simulink model "Simulate_motor_controllers"  (R2014b)
settings: Solver=ode45  SolverMode=SingleTasking  StartTime=0.0  StopTime=5  RelTol=1e-3
values from neighbouring files (symbols this model uses):
  D = abs((2*J^2*zeta*omega*r^2+J^2*omega2*r^2-J*d*r^2+d^2*r^2-J*k*r+2*d*k*r+k^2)/(k*(J*r-d*r-k)))    [workshop1.m]
  enable_karnop = 0    [workshop1.m]
  enable_sin = 0    [workshop1.m]
  F_c = 0.0008    [workshop1.m]
  I = abs(omega^2*omega2*J^2*r^2/((J*r-d*r-k)*k))    [workshop1.m]
  J = Jtot    (= 2.22222222222e-05)    [workshop1.m]
  Jtot = 1/45000    (= 2.22222222222e-05)    [workshop1.m]
  motor = motor_pars    [workshop1.m]
  n = 5    [workshop1.m]
  P = abs(J^2*omega*r^2*(2*zeta*omega2+omega)/(k*(J*r-d*r-k)))    [workshop1.m]
  R = s*(1+r0*s)    [workshop1.m]
  r0 = abs(J*r/(J*r-d*r-k))    [workshop1.m]
  S = P*s+D*s^2+I    [workshop1.m]
  sim_sin_amp = 1    [workshop1.m]
  sim_sin_freq = 1    [workshop1.m]
  T = P*s+D*s^2+I    [workshop1.m]
  Ts = 0.002    [workshop1.m]
libraries: simulink x5
settings Model: Creator=Gabriel  LastModifiedBy=es2lab2
settings OptimizationCC: BlockReduction=off  BooleanDataType=off
settings DebuggingCC: SaveWithParameterizedLinksMsg=none  UnderspecifiedInitializationDetection=Classic  MergeDetectMultiDrivingBlocksExec=none  SignalResolutionControl=TryResolveAllWithWarning  SolverPrmCheckMsg=none
settings HardwareCC: TargetIntDivRoundTo=Zero  TargetEndianess=LittleEndian  TargetHWDeviceType=MATLAB Host  ProdEqTarget=off

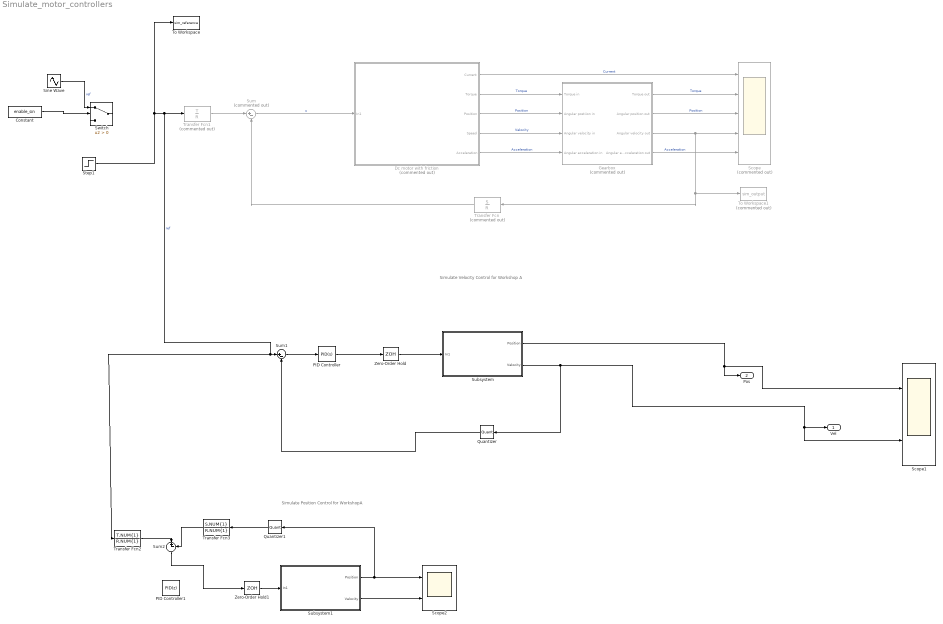
== system Simulate_motor_controllers ==
  note: Simulate Position Control for WorkshopA
  note: Simulate Velocity Control for Workshop A
  Constant : Constant  Value=enable_sin
  Dc motor with friction : Subsystem  Commented=on
      mask Display:
      | image('dcmotor.jpg')
      | port_label('input', 1, 'Voltage')
      | port_label('output', 1, 'Current')
      | port_label('output', 2, 'Torque')
      | port_label('output', 3, 'Position')
      | port_label('output', 4, 'Velocity')
      | port_label('output', 5, 'Acceleration')
  Gearbox : Subsystem  Commented=on
  PID Controller : simulink/Continuous/PID Controller  Controller=PID  TimeDomain=Continuous-time  SampleTime=-1  IntegratorMethod=Forward Euler  FilterMethod=Forward Euler  Form=Parallel  P=P  I=I  D=0  N=100  InitialConditionSource=internal  InitialConditionForIntegrator=0  InitialConditionForFilter=0  ExternalReset=none  LimitOutput=off  UpperSaturationLimit=inf  LowerSaturationLimit=-inf  LinearizeAsGain=on  AntiWindupMode=none  Kb=1  TrackingMode=off  Kt=1  PParamMin=[]  PParamMax=[]  IParamMin=[]  IParamMax=[]  DParamMin=[]  DParamMax=[]  NParamMin=[]  NParamMax=[]  KbParamMin=[]  KbParamMax=[]  KtParamMin=[]  KtParamMax=[]  POutMin=[]  POutMax=[]  IOutMin=[]  IOutMax=[]  DOutMin=[]  DOutMax=[]  NOutMin=[]  NOutMax=[]  KbOutMin=[]  KbOutMax=[]  KtOutMin=[]  KtOutMax=[]  IntegratorOutMin=[]  IntegratorOutMax=[]  FilterOutMin=[]  FilterOutMax=[]  SumOutMin=[]  SumOutMax=[]  SumI1OutMin=[]  SumI1OutMax=[]  SumI2OutMin=[]  SumI2OutMax=[]  SumI3OutMin=[]  SumI3OutMax=[]  SumDOutMin=[]  SumDOutMax=[]  SaturationOutMin=[]  SaturationOutMax=[]  IntegratorContinuousStateAttributes=''  IntegratorStateMustResolveToSignalObject=off  IntegratorRTWStateStorageClass=Auto  FilterContinuousStateAttributes=''  FilterStateMustResolveToSignalObject=off  FilterRTWStateStorageClass=Auto  DifferentiatorICPrevScaledInput=0  DifferentiatorOutMin=[]  DifferentiatorOutMax=[]  UseFilter=on
  PID Controller1 : simulink/Continuous/PID Controller  Controller=PID  TimeDomain=Discrete-time  SampleTime=Ts  IntegratorMethod=Forward Euler  FilterMethod=Forward Euler  Form=Parallel  P=P  I=I  D=D  N=r0  InitialConditionSource=internal  InitialConditionForIntegrator=0  InitialConditionForFilter=0  ExternalReset=none  LimitOutput=off  UpperSaturationLimit=inf  LowerSaturationLimit=-inf  LinearizeAsGain=on  AntiWindupMode=none  Kb=1  TrackingMode=off  Kt=1  PParamMin=[]  PParamMax=[]  IParamMin=[]  IParamMax=[]  DParamMin=[]  DParamMax=[]  NParamMin=[]  NParamMax=[]  KbParamMin=[]  KbParamMax=[]  KtParamMin=[]  KtParamMax=[]  POutMin=[]  POutMax=[]  IOutMin=[]  IOutMax=[]  DOutMin=[]  DOutMax=[]  NOutMin=[]  NOutMax=[]  KbOutMin=[]  KbOutMax=[]  KtOutMin=[]  KtOutMax=[]  IntegratorOutMin=[]  IntegratorOutMax=[]  FilterOutMin=[]  FilterOutMax=[]  SumOutMin=[]  SumOutMax=[]  SumI1OutMin=[]  SumI1OutMax=[]  SumI2OutMin=[]  SumI2OutMax=[]  SumI3OutMin=[]  SumI3OutMax=[]  SumDOutMin=[]  SumDOutMax=[]  SaturationOutMin=[]  SaturationOutMax=[]  IntegratorContinuousStateAttributes=''  IntegratorStateMustResolveToSignalObject=off  IntegratorRTWStateStorageClass=Auto  FilterContinuousStateAttributes=''  FilterStateMustResolveToSignalObject=off  FilterRTWStateStorageClass=Auto  DifferentiatorICPrevScaledInput=0  DifferentiatorOutMin=[]  DifferentiatorOutMax=[]  UseFilter=on
  Quantizer : Quantizer  QuantizationInterval=Ts
  Quantizer1 : Quantizer  QuantizationInterval=Ts
  Scope : Scope  Commented=on  NumInputPorts=5
      settings: YMin=-0.7198~-0.25085~-1.49914~-4.86523~-4731.78811~-16.47182~-16.47182~-16.47182  YMax=1.13271~0.39475~13.49228~43.78709~7102.06049~16.47182~16.47182~16.47182
  Scope1 : Scope  NumInputPorts=2
      settings: YMin=-2.5e-06~-0.0001  YMax=0~2e-05
  Scope2 : Scope  NumInputPorts=2
      settings: TimeRange=5  YMin=0~-10  YMax=4.5~60  SaveName=ScopeData2
  Sine Wave : Sin  Amplitude=sim_sin_amp  Frequency=sim_sin_freq  SampleTime=0
  Step1 : Step  Time=0  After=4  SampleTime=0
  Subsystem : Subsystem
  Subsystem1 : Subsystem
  Sum : Sum  Commented=on  Inputs=|+-
  Sum1 : Sum  Inputs=|+-
  Sum2 : Sum  Inputs=|+-
  Switch : Switch  Criteria=u2 > Threshold
  To Workspace : ToWorkspace  VariableName=sim_reference  SaveFormat=Timeseries  SampleTime=-1
  To Workspace1 : ToWorkspace  Commented=on  VariableName=sim_output  SaveFormat=Timeseries  SampleTime=-1
  Transfer Fcn : TransferFcn  Commented=on  Numerator=S  Denominator=R
  Transfer Fcn1 : TransferFcn  Commented=on  Numerator=T  Denominator=R
  Transfer Fcn2 : TransferFcn  Numerator=T.NUM{1}  Denominator=R.NUM{1}
  Transfer Fcn3 : TransferFcn  Numerator=S.NUM{1}  Denominator=R.NUM{1}
  Zero-Order Hold : ZeroOrderHold  SampleTime=Ts
  Zero-Order Hold1 : ZeroOrderHold  SampleTime=Ts
  Vel : Outport
  Pos : Outport  Port=2
  wires:
  Constant/1 -> Switch/2
  Dc motor with friction/4(Speed) -> Gearbox/3(Angular velocity in)  "Velocity"
  Dc motor with friction/2(Torque) -> Gearbox/1(Torque in)  "Torque"
  Dc motor with friction/1(Current) -> Scope/1  "Current"
  Dc motor with friction/5(Acceleration) -> Gearbox/4(Angular acceleration in)  "Acceleration"
  Dc motor with friction/3(Position) -> Gearbox/2(Angular postiion in)  "Position"
  Gearbox/1(Torque out) -> Scope/2  "Torque"
  Gearbox/2(Angular position out) -> Scope/3  "Position"
  Gearbox/3(Angular velocity out) -> Transfer Fcn/1, To Workspace1/1, Scope/4
  Gearbox/4(Angular acceleration out) -> Scope/5  "Acceleration"
  Transfer Fcn/1 -> Sum/2
  Transfer Fcn1/1 -> Sum/1
  Sum/1 -> Dc motor with friction/1(In1)  "u"
  Subsystem/1(Position) -> Pos/1, Scope1/1
  Subsystem/2(Velocity) -> Quantizer/1, Vel/1, Scope1/2
  Sum1/1 -> PID Controller/1
  Zero-Order Hold/1 -> Subsystem/1(In1)
  Quantizer/1 -> Sum1/2
  PID Controller/1 -> Zero-Order Hold/1
  Step1/1 -> Transfer Fcn2/1, Sum1/1, Transfer Fcn1/1, To Workspace/1  "ref"
  Subsystem1/1(Position) -> Quantizer1/1, Scope2/1
  Subsystem1/2(Velocity) -> Scope2/2
  Zero-Order Hold1/1 -> Subsystem1/1(In1)
  Transfer Fcn3/1 -> Sum2/2
  Sine Wave/1 -> Switch/1  "ref"
  Sum2/1 -> Zero-Order Hold1/1
  Transfer Fcn2/1 -> Sum2/1
  Quantizer1/1 -> Transfer Fcn3/1

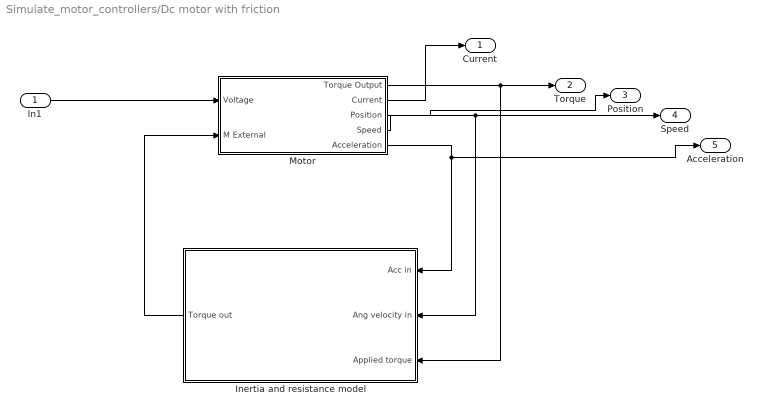
== system Simulate_motor_controllers/Dc motor with friction ==
  In1 : Inport
  "Inertia and resistance model " : Subsystem
  Motor : Subsystem
  Current : Outport
  Torque : Outport  Port=2
  Position : Outport  Port=3
  Speed : Outport  Port=4
  Acceleration : Outport  Port=5
  wires:
  Motor/4(Speed) -> Speed/1, "Inertia and resistance model "/2(Ang velocity in)
  Motor/3(Position) -> Position/1
  Motor/2(Current) -> Current/1
  "Inertia and resistance model "/1(Torque out) -> Motor/2("M External ")
  Motor/1(Torque Output) -> Torque/1, "Inertia and resistance model "/3(Applied torque)
  In1/1 -> Motor/1(Voltage)
  Motor/5(Acceleration) -> "Inertia and resistance model "/1(Acc in), Acceleration/1

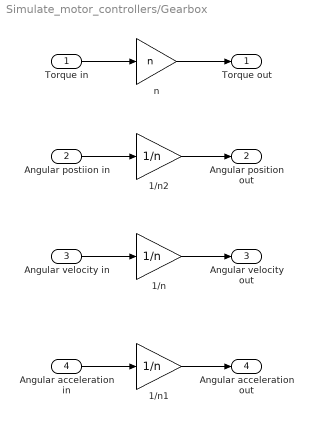
== system Simulate_motor_controllers/Gearbox ==
  Torque in : Inport
  Angular postiion in : Inport  Port=2
  Angular velocity in : Inport  Port=3
  Angular acceleration in : Inport  Port=4
  1/n : Gain  Gain=1/n
  1/n1 : Gain  Gain=1/n
  1/n2 : Gain  Gain=1/n
  n : Gain  Gain=n
  Torque out : Outport
  Angular position out : Outport  Port=2
  Angular velocity out : Outport  Port=3
  Angular acceleration out : Outport  Port=4
  wires:
  1/n/1 -> Angular velocity out/1
  Angular velocity in/1 -> 1/n/1
  n/1 -> Torque out/1
  Torque in/1 -> n/1
  1/n1/1 -> Angular acceleration out/1
  Angular acceleration in/1 -> 1/n1/1
  1/n2/1 -> Angular position out/1
  Angular postiion in/1 -> 1/n2/1

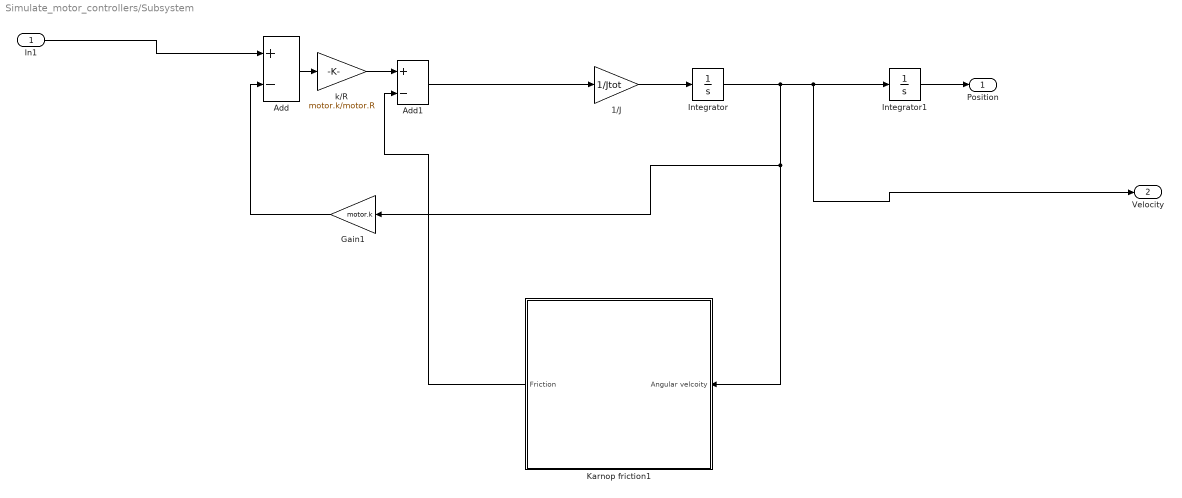
== system Simulate_motor_controllers/Subsystem ==
  In1 : Inport
  1/J : Gain  Gain=1/Jtot
  Add : Sum  Inputs=+-
  Add1 : Sum  Inputs=+-
  Gain1 : Gain  Gain=motor.k
  Integrator : Integrator
  Integrator1 : Integrator
  Karnop friction1 : Subsystem
  "k/R " : Gain  Gain=motor.k/motor.R
  Position : Outport
  Velocity : Outport  Port=2
  wires:
  In1/1 -> Add/1
  Add1/1 -> 1/J/1
  Karnop friction1/1(Friction) -> Add1/2
  Integrator1/1 -> Position/1
  Integrator/1 -> Karnop friction1/1(Angular velcoity), Gain1/1, Velocity/1, Integrator1/1
  1/J/1 -> Integrator/1
  "k/R "/1 -> Add1/1
  Add/1 -> "k/R "/1
  Gain1/1 -> Add/2

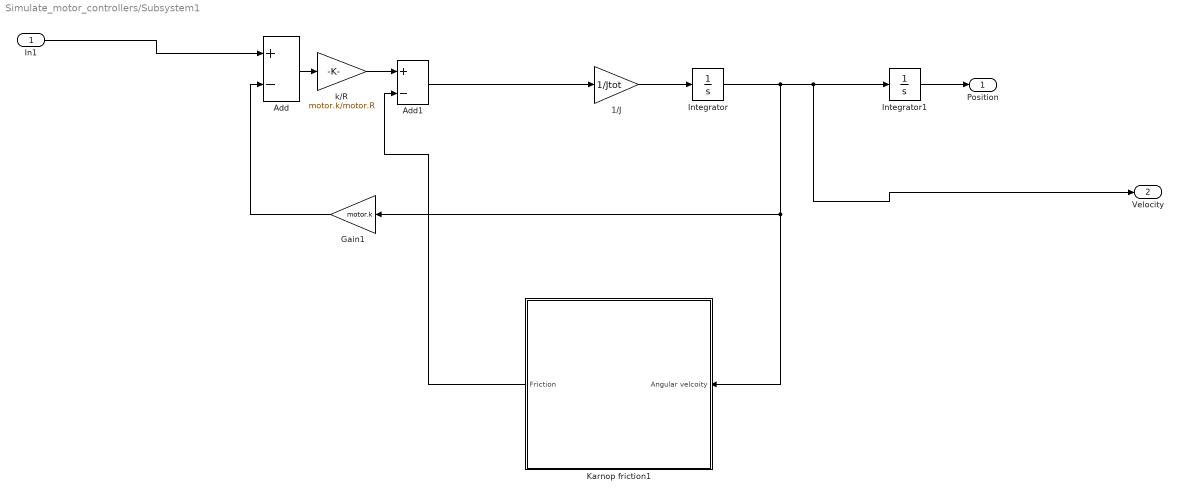
== system Simulate_motor_controllers/Subsystem1 ==
  In1 : Inport
  1/J : Gain  Gain=1/Jtot
  Add : Sum  Inputs=+-
  Add1 : Sum  Inputs=+-
  Gain1 : Gain  Gain=motor.k
  Integrator : Integrator
  Integrator1 : Integrator
  Karnop friction1 : Subsystem
  "k/R " : Gain  Gain=motor.k/motor.R
  Position : Outport
  Velocity : Outport  Port=2
  wires:
  Gain1/1 -> Add/2
  Add/1 -> "k/R "/1
  "k/R "/1 -> Add1/1
  1/J/1 -> Integrator/1
  Integrator/1 -> Integrator1/1, Velocity/1, Gain1/1, Karnop friction1/1(Angular velcoity)
  Integrator1/1 -> Position/1
  Karnop friction1/1(Friction) -> Add1/2
  Add1/1 -> 1/J/1
  In1/1 -> Add/1

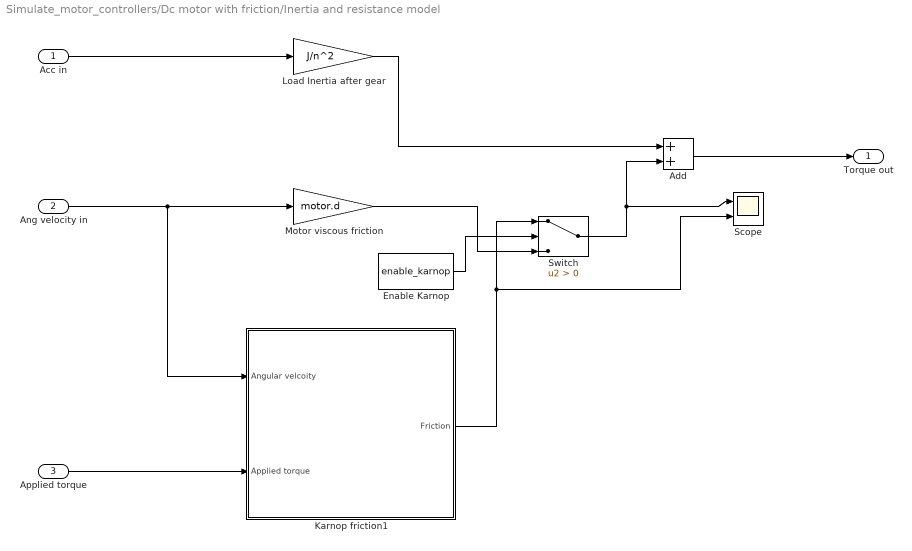
== system Simulate_motor_controllers/Dc motor with friction/Inertia and resistance model  ==
  Acc in : Inport
  Ang velocity in : Inport  Port=2
  Applied torque : Inport  Port=3
  Add : Sum
  Enable Karnop : Constant  Value=enable_karnop
  Karnop friction1 : Subsystem
  Load Inertia after gear : Gain  Gain=J/n^2
  Motor viscous friction : Gain  Gain=motor.d
  Scope : Scope  NumInputPorts=2
      settings: YMin=-0.00177~-0.00177  YMax=0.00177~0.00177
  Switch : Switch  Criteria=u2 > Threshold
  Torque out : Outport
  wires:
  Acc in/1 -> Load Inertia after gear/1
  Add/1 -> Torque out/1
  Load Inertia after gear/1 -> Add/1
  Ang velocity in/1 -> Karnop friction1/1(Angular velcoity), Motor viscous friction/1
  Motor viscous friction/1 -> Switch/3
  Karnop friction1/1(Friction) -> Switch/1, Scope/2
  Switch/1 -> Add/2, Scope/1
  Enable Karnop/1 -> Switch/2
  Applied torque/1 -> Karnop friction1/2("Applied torque ")

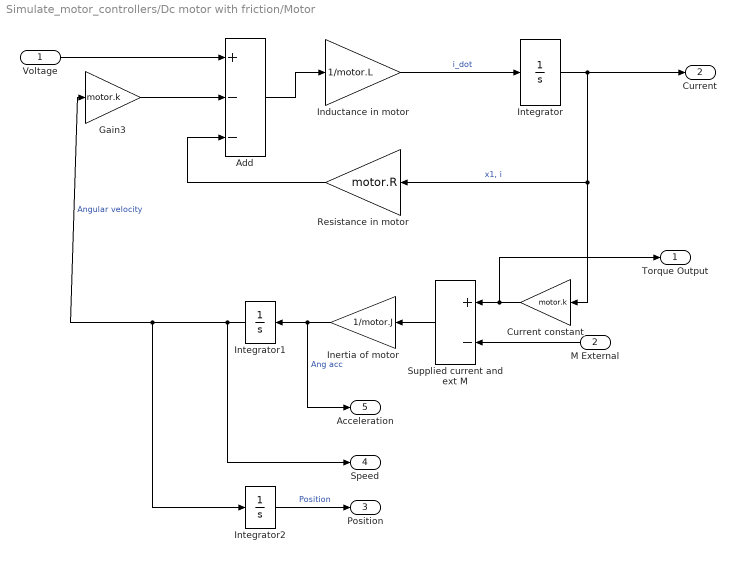
== system Simulate_motor_controllers/Dc motor with friction/Motor ==
  Voltage : Inport
  "M External " : Inport  Port=2
  Add : Sum  Inputs=+--
  Current constant : Gain  Gain=motor.k
  Gain3 : Gain  Gain=motor.k
  Inductance in motor : Gain  Gain=1/motor.L
  Inertia of motor : Gain  Gain=1/motor.J
  Integrator : Integrator
  Integrator1 : Integrator
  Integrator2 : Integrator
  Resistance in motor : Gain  Gain=motor.R
  "Supplied current and ext M " : Sum  Inputs=+-
  Torque Output : Outport
  Current : Outport  Port=2
  Position : Outport  Port=3
  Speed : Outport  Port=4
  Acceleration : Outport  Port=5
  wires:
  Voltage/1 -> Add/1
  Add/1 -> Inductance in motor/1
  Inductance in motor/1 -> Integrator/1  "i_dot"
  Integrator/1 -> Current constant/1, Resistance in motor/1, Current/1  "x1, i"
  Resistance in motor/1 -> Add/3
  Gain3/1 -> Add/2
  Integrator1/1 -> Speed/1, Integrator2/1, Gain3/1  "Angular velocity"
  "Supplied current and ext M "/1 -> Inertia of motor/1
  Inertia of motor/1 -> Acceleration/1, Integrator1/1  "Ang acc"
  Current constant/1 -> Torque Output/1, "Supplied current and ext M "/1
  "M External "/1 -> "Supplied current and ext M "/2
  Integrator2/1 -> Position/1  "Position"

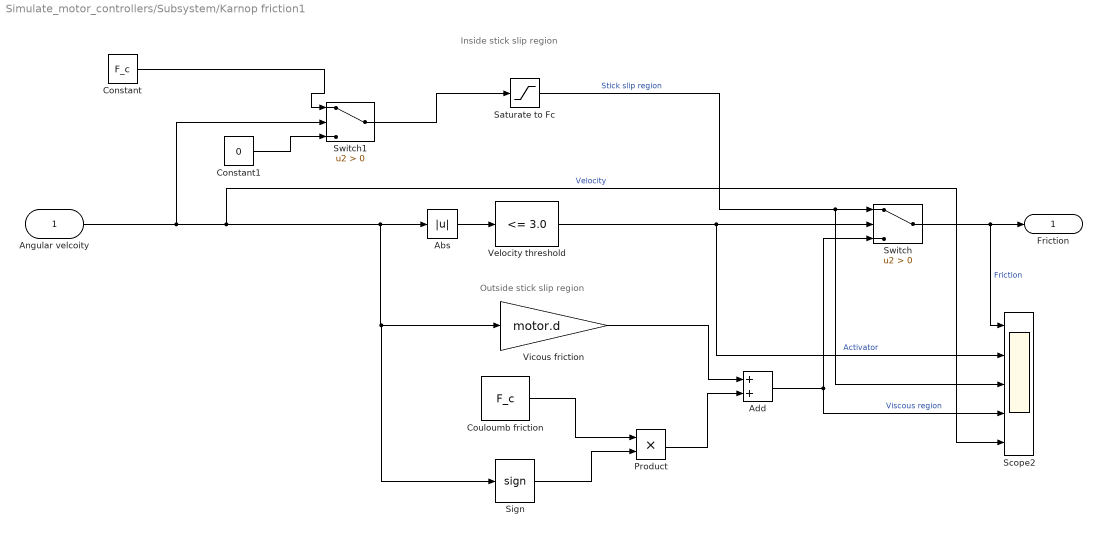
== system Simulate_motor_controllers/Subsystem/Karnop friction1 ==
  note: Outside stick slip region
  note: Inside stick slip region
  Angular velcoity : Inport
  Abs : Abs  ZeroCross=off
  Add : Sum
  Constant : Constant  Value=F_c
  Constant1 : Constant  Value=0
  Couloumb friction : Constant  Value=F_c
  Product : Product
  Saturate to Fc : Saturate  UpperLimit=F_c  LowerLimit=-F_c  ZeroCross=off
  Scope2 : Scope  NumInputPorts=5
      settings: ShowLegends=on  YMin=-0.00177~-0.125~0.0009~-0.00177~-138.1533~-0.12501~-0.12501~-0.12501  YMax=0.00177~1.125~0.0011~0.00177~138.10681~0.12501~0.12501~0.12501  SaveName=ScopeData3
  Sign : Signum  ZeroCross=off
  Switch : Switch  Criteria=u2 > Threshold  ZeroCross=off
  Switch1 : Switch  Criteria=u2 > Threshold  ZeroCross=off
  "Velocity threshold " : simulink/Logic and Bit Operations/Compare To Constant  relop=<=  const=3.0  OutDataTypeStr=boolean
  Vicous friction : Gain  Gain=motor.d
  Friction : Outport
  wires:
  Add/1 -> Scope2/4, Switch/3  "Viscous region"
  Sign/1 -> Product/2
  Couloumb friction/1 -> Product/1
  Vicous friction/1 -> Add/1
  Product/1 -> Add/2
  Abs/1 -> "Velocity threshold "/1
  "Velocity threshold "/1 -> Switch/2, Scope2/2  "Activator"
  Angular velcoity/1 -> Switch1/2, Sign/1, Vicous friction/1, Abs/1, Scope2/5  "Velocity"
  Switch/1 -> Friction/1, Scope2/1  "Friction"
  Saturate to Fc/1 -> Switch/1, Scope2/3  "Stick slip region"
  Constant/1 -> Switch1/1
  Constant1/1 -> Switch1/3
  Switch1/1 -> Saturate to Fc/1

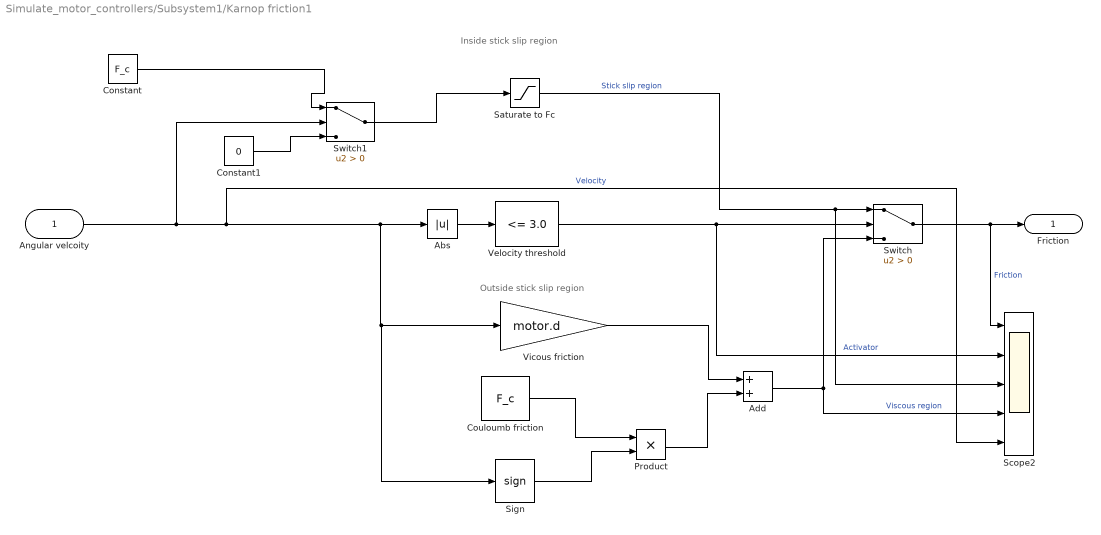
== system Simulate_motor_controllers/Subsystem1/Karnop friction1 ==
  note: Inside stick slip region
  note: Outside stick slip region
  Angular velcoity : Inport
  Abs : Abs  ZeroCross=off
  Add : Sum
  Constant : Constant  Value=F_c
  Constant1 : Constant  Value=0
  Couloumb friction : Constant  Value=F_c
  Product : Product
  Saturate to Fc : Saturate  UpperLimit=F_c  LowerLimit=-F_c  ZeroCross=off
  Scope2 : Scope  NumInputPorts=5
      settings: ShowLegends=on  YMin=-0.00177~-0.125~0.0009~-0.00177~-138.153  YMax=0.00177~1.125~0.0011~0.00177~138.107  SaveName=ScopeData3
  Sign : Signum  ZeroCross=off
  Switch : Switch  Criteria=u2 > Threshold  ZeroCross=off
  Switch1 : Switch  Criteria=u2 > Threshold  ZeroCross=off
  "Velocity threshold " : simulink/Logic and Bit Operations/Compare To Constant  relop=<=  const=3.0  OutDataTypeStr=boolean  ZeroCross=off
  Vicous friction : Gain  Gain=motor.d
  Friction : Outport
  wires:
  Switch1/1 -> Saturate to Fc/1
  Constant1/1 -> Switch1/3
  Constant/1 -> Switch1/1
  Saturate to Fc/1 -> Scope2/3, Switch/1  "Stick slip region"
  Switch/1 -> Scope2/1, Friction/1  "Friction"
  Angular velcoity/1 -> Scope2/5, Abs/1, Vicous friction/1, Sign/1, Switch1/2  "Velocity"
  "Velocity threshold "/1 -> Scope2/2, Switch/2  "Activator"
  Abs/1 -> "Velocity threshold "/1
  Product/1 -> Add/2
  Vicous friction/1 -> Add/1
  Couloumb friction/1 -> Product/1
  Sign/1 -> Product/2
  Add/1 -> Switch/3, Scope2/4  "Viscous region"

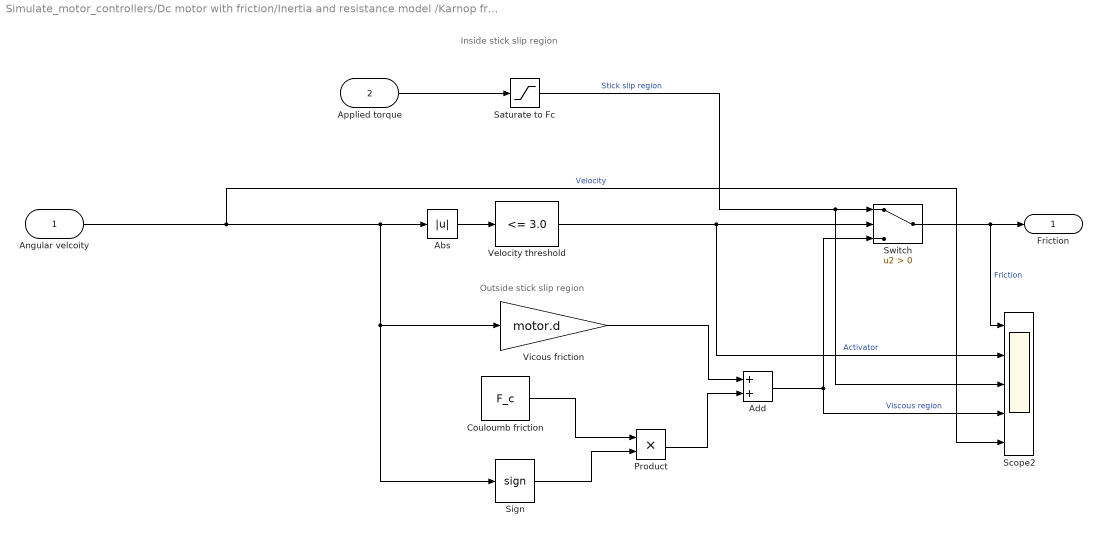
== system Simulate_motor_controllers/Dc motor with friction/Inertia and resistance model /Karnop friction1 ==
  note: Inside stick slip region
  note: Outside stick slip region
  Angular velcoity : Inport
  "Applied torque " : Inport  Port=2
  Abs : Abs
  Add : Sum
  Couloumb friction : Constant  Value=F_c
  Product : Product
  Saturate to Fc : Saturate  UpperLimit=F_c  LowerLimit=-F_c
  Scope2 : Scope  NumInputPorts=5
      settings: ShowLegends=on  YMin=-0.00177~-0.125~0.0009~-0.00177~-138.1533~-0.12501~-0.12501~-0.12501  YMax=0.00177~1.125~0.0011~0.00177~138.10681~0.12501~0.12501~0.12501  SaveName=ScopeData3
  Sign : Signum
  Switch : Switch  Criteria=u2 > Threshold
  "Velocity threshold " : simulink/Logic and Bit Operations/Compare To Constant  relop=<=  const=3.0  OutDataTypeStr=boolean
  Vicous friction : Gain  Gain=motor.d
  Friction : Outport
  wires:
  Saturate to Fc/1 -> Scope2/3, Switch/1  "Stick slip region"
  Switch/1 -> Scope2/1, Friction/1  "Friction"
  Angular velcoity/1 -> Scope2/5, Abs/1, Vicous friction/1, Sign/1  "Velocity"
  "Velocity threshold "/1 -> Scope2/2, Switch/2  "Activator"
  Abs/1 -> "Velocity threshold "/1
  Product/1 -> Add/2
  Vicous friction/1 -> Add/1
  Couloumb friction/1 -> Product/1
  Sign/1 -> Product/2
  "Applied torque "/1 -> Saturate to Fc/1
  Add/1 -> Switch/3, Scope2/4  "Viscous region"
